simulink model "sampleModel1762_5_sub_sub"  (R2023a)
settings: Solver=VariableStepAuto  StartTime=0.0  StopTime=10.0  RelTol=1e-3
libraries: hdlsllib x1
settings Model: Creator=user1  LastModifiedBy=user1

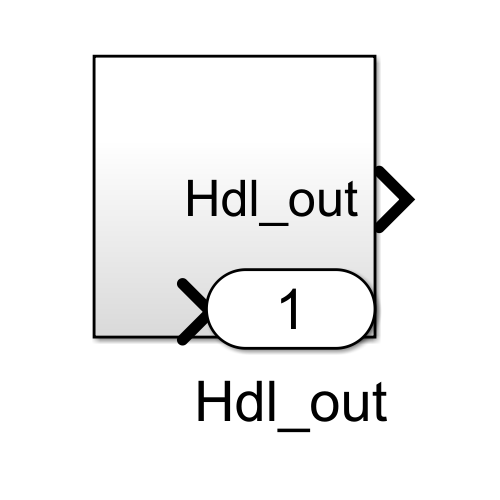
[thumbnail: Simulink's stored preview of the top-level diagram]
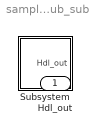
== system sampleModel1762_5_sub_sub ==
  Subsystem : Subsystem
  Hdl_out : Outport  OutDataTypeStr=uint8

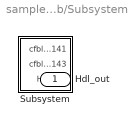
== system sampleModel1762_5_sub_sub/Subsystem ==
  Subsystem : Subsystem
  Hdl_out : Outport  OutDataTypeStr=uint8

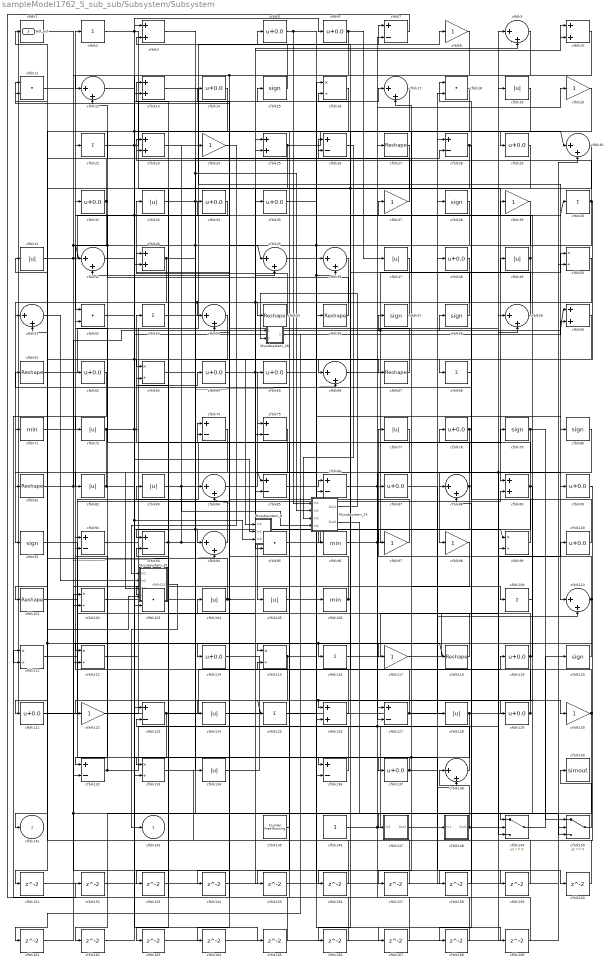
== system sampleModel1762_5_sub_sub/Subsystem/Subsystem ==
  Mysubsystem_23 : Subsystem  TreatAsAtomicUnit=on  RTWFcnName=Mysubsystem_23
      settings: RTWFcnNameOpts=User specified  RTWFileNameOpts=Use function name
  Mysubsystem_28 : Subsystem  TreatAsAtomicUnit=on  RTWFcnName=Mysubsystem_28
      settings: RTWFcnNameOpts=User specified  RTWFileNameOpts=Use function name
  Mysubsystem_35 : Subsystem  TreatAsAtomicUnit=on  RTWFcnName=Mysubsystem_35
      settings: RTWFcnNameOpts=User specified  RTWFileNameOpts=Use function name
  Mysubsystem_8 : Subsystem  TreatAsAtomicUnit=on  RTWFcnName=Mysubsystem_8
      settings: RTWFcnNameOpts=User specified  RTWFileNameOpts=Use function name
  cfblk{1,71,96,106} (4 alike) : MinMax  OutDataTypeStr=uint8
  cfblk{3,10,13,23,25,43,60,89,126} (9 alike) : Sum  OutDataTypeStr=uint8
  cfblk{5..6,14,29,32,34..35,48,62,64..65,78,87,90,100,114,119,121,129,137} (20 alike) : Bias  Bias=0.0  SaturateOnIntegerOverflow=off
  cfblk{27,55..56,61,67,81,101,118} (8 alike) : Reshape
  cfblk{16,50,63,99,102,111..112,115,133} (9 alike) : Product  Inputs=*/  OutDataTypeStr=uint8  RndMeth=Zero  SaturateOnIntegerOverflow=on
  cfblk{11,18,52,95,103} (5 alike) : DotProduct  OutDataTypeStr=uint8
  cfblk{19,33,41,47,49,72,77,82..83,104..105,124,128,134} (14 alike) : Abs  OutDataTypeStr=uint8  SaturateOnIntegerOverflow=off
  cfblk{2,22,40,53,68,109,116,125} (8 alike) : Sum  Inputs=+  OutDataTypeStr=uint8
  cfblk{9,12,17,30,42,45..46,51,54,59,66,84,88,94,110,138} (16 alike) : Sum  Inputs=|++  OutDataTypeStr=uint8
  cfblk{8,20,24,37,39,97..98,117,122,130} (10 alike) : Gain  OutDataTypeStr=uint8
  cfblk{15,38,57..58,79..80,91,120} (8 alike) : Signum
  cfblk{7,26,28,74..75,85..86,92..93,123,127,132,136} (13 alike) : Sum  Inputs=+-  OutDataTypeStr=uint8
  cfblk140 : ToWorkspace  VariableName=simout  SaveFormat=Timeseries  SampleTime=-1
  cfblk145 : hdlsllib/Sources/Counter Free-Running  NumBits=16  tsamp=-1
  cfblk146 : Constant  OutDataTypeStr=uint8  SampleTime=-1
  cfblk147 : Subsystem
      settings: LibrarySourceBlock=|
      | hdlsllib/Ports &
      | Subsystems/Subsystem
  cfblk148 : Subsystem
      settings: LibrarySourceBlock=|
      | hdlsllib/Ports &
      | Subsystems/Subsystem
  cfblk149 : Switch  OutDataTypeStr=uint8  SaturateOnIntegerOverflow=off  InputSameDT=off
  cfblk150 : Switch  OutDataTypeStr=uint8  SaturateOnIntegerOverflow=off  InputSameDT=off
  cfblk{151..169} (19 alike) : Delay  SampleTime=1
  cfblk141 : Outport  OutDataTypeStr=uint8  VectorParamsAs1DForOutWhenUnconnected=off
  cfblk143 : Outport  Port=2  OutDataTypeStr=uint8  VectorParamsAs1DForOutWhenUnconnected=off
  Hdl_out : Outport  Port=3  OutDataTypeStr=uint8
  wires:
  Mysubsystem_35/1(cfblk143) -> cfblk143/1
  cfblk77/1 -> Mysubsystem_35/3(In3)
  cfblk51/1 -> Mysubsystem_35/2(In2)
  cfblk24/1 -> Mysubsystem_35/1(In1)
  Mysubsystem_28/1(Out1) -> cfblk161/1
  Mysubsystem_23/1(Out1) -> Mysubsystem_28/2(In2)
  Mysubsystem_23/2(Out2) -> cfblk162/1
  cfblk26/1 -> Mysubsystem_23/3(In3)
  cfblk52/1 -> Mysubsystem_8/2(In2)
  cfblk169/1 -> cfblk111/1
  cfblk65/1 -> cfblk169/1
  cfblk168/1 -> cfblk127/1
  cfblk39/1 -> cfblk168/1
  cfblk167/1 -> cfblk93/2
  cfblk125/1 -> cfblk167/1
  cfblk166/1 -> cfblk115/2
  cfblk165/1 -> cfblk54/2
  cfblk164/1 -> cfblk30/2
  cfblk163/1 -> cfblk99/2
  cfblk162/1 -> cfblk123/1
  cfblk161/1 -> cfblk102/1
  cfblk160/1 -> cfblk28/1
  cfblk159/1 -> cfblk3/1
  cfblk158/1 -> cfblk88/2
  cfblk157/1 -> cfblk1/1
  cfblk156/1 -> cfblk25/1
  cfblk155/1 -> cfblk138/2
  cfblk38/1 -> cfblk155/1
  cfblk154/1 -> cfblk46/1
  cfblk153/1 -> cfblk50/2
  cfblk29/1 -> cfblk153/1
  cfblk152/1 -> cfblk85/2
  cfblk7/1 -> cfblk152/1
  cfblk151/1 -> cfblk18/2
  cfblk5/1 -> Mysubsystem_23/1(In1), cfblk130/1
  cfblk15/1 -> cfblk5/1
  cfblk14/1 -> cfblk51/2
  cfblk124/1 -> cfblk106/1
  cfblk37/1 -> cfblk12/2
  cfblk12/1 -> cfblk95/1, Mysubsystem_8/3(In3), cfblk30/1
  cfblk98/1 -> cfblk117/1
  cfblk58/1 -> cfblk17/2
  cfblk8/1 -> cfblk43/2
  cfblk119/1 -> cfblk125/1, cfblk126/1, cfblk23/1, cfblk39/1
  cfblk60/1 -> cfblk112/1
  cfblk129/1 -> cfblk14/1, Hdl_out/1
  cfblk56/1 -> cfblk32/1
  cfblk74/1 -> cfblk141/1
  cfblk6/1 -> cfblk12/1, cfblk47/1
  cfblk49/1 -> cfblk54/1, cfblk103/1, cfblk26/2
  cfblk103/1 -> cfblk58/1
  cfblk45/1 -> cfblk80/1
  cfblk63/1 -> cfblk99/1, cfblk149/2
  cfblk78/1 -> cfblk18/1, cfblk127/2
  cfblk133/1 -> cfblk57/1
  cfblk93/1 -> cfblk84/1, cfblk26/1, cfblk63/2
  cfblk111/1 -> cfblk35/1
  cfblk28/1 -> cfblk68/1, cfblk95/2
  cfblk67/1 -> cfblk11/1
  cfblk101/1 -> cfblk25/2
  cfblk117/1 -> cfblk19/1
  cfblk116/1 -> cfblk59/2
  cfblk130/1 -> cfblk16/2, cfblk163/1
  cfblk71/1 -> cfblk62/1
  cfblk64/1 -> cfblk86/2, cfblk10/1
  cfblk50/1 -> cfblk55/1
  cfblk30/1 -> cfblk124/1
  cfblk81/1 -> Mysubsystem_28/1(In1), cfblk109/1
  cfblk68/1 -> cfblk88/1
  cfblk115/1 -> cfblk28/2, cfblk122/1
  cfblk118/1 -> cfblk83/1
  cfblk82/1 -> cfblk81/1, cfblk94/1
  cfblk46/1 -> cfblk93/1, cfblk75/2
  cfblk145/1 -> cfblk75/1
  cfblk47/1 -> cfblk121/1
  cfblk62/1 -> cfblk111/2
  cfblk43/1 -> cfblk132/2, cfblk137/1
  cfblk112/1 -> cfblk74/2
  cfblk80/1 -> cfblk85/1, cfblk149/3
  cfblk85/1 -> cfblk86/1
  cfblk84/1 -> cfblk65/1
  cfblk128/1 -> cfblk156/1, cfblk157/1, cfblk158/1
  cfblk121/1 -> cfblk89/2
  cfblk10/1 -> cfblk13/2
  cfblk42/1 -> cfblk15/1, cfblk40/1
  cfblk19/1 -> cfblk147/1(In1)
  cfblk22/1 -> cfblk8/1, cfblk165/1
  cfblk147/1(Out1) -> cfblk110/2
  cfblk94/1 -> cfblk13/1
  cfblk90/1 -> cfblk134/1
  cfblk127/1 -> cfblk50/1, cfblk92/1
  cfblk105/1 -> cfblk16/1
  cfblk91/1 -> cfblk148/1(In1)
  cfblk16/1 -> cfblk132/1
  cfblk3/1 -> cfblk45/1, cfblk67/1
  cfblk40/1 -> Mysubsystem_8/1(In1), cfblk126/2, cfblk164/1, cfblk23/2
  cfblk27/1 -> cfblk63/1, cfblk136/1
  cfblk53/1 -> cfblk7/2
  cfblk123/1 -> cfblk48/1, cfblk133/2
  cfblk132/1 -> cfblk38/1, cfblk87/1, cfblk92/2
  cfblk109/1 -> cfblk149/1
  cfblk99/1 -> cfblk61/1
  cfblk86/1 -> cfblk78/1, cfblk90/1
  cfblk92/1 -> cfblk56/1
  cfblk136/1 -> cfblk123/2
  cfblk79/1 -> cfblk98/1, cfblk150/1
  cfblk95/1 -> cfblk97/1
  cfblk106/1 -> cfblk42/2, cfblk166/1
  cfblk1/1 -> cfblk116/1, cfblk118/1, cfblk45/2
  cfblk104/1 -> cfblk9/2, cfblk84/2, cfblk41/1
  cfblk66/1 -> cfblk60/1, cfblk10/2
  cfblk146/1 -> cfblk59/1, cfblk20/1
  cfblk61/1 -> cfblk9/1
  cfblk150/1 -> cfblk140/1
  cfblk20/1 -> cfblk42/1, cfblk72/1
  cfblk23/1 -> Mysubsystem_23/2(In2), cfblk66/2
  cfblk54/1 -> cfblk101/1, cfblk103/2
  cfblk138/1 -> cfblk104/1
  cfblk35/1 -> cfblk46/2, cfblk150/2
  cfblk120/1 -> cfblk114/1
  cfblk148/1(Out1) -> cfblk138/1, cfblk100/1
  cfblk75/1 -> cfblk82/1
  cfblk41/1 -> cfblk34/1, cfblk94/2
  cfblk72/1 -> cfblk64/1, cfblk60/2, cfblk112/2
  cfblk97/1 -> cfblk43/1
  cfblk18/1 -> cfblk66/1
  cfblk87/1 -> cfblk128/1
  cfblk83/1 -> Mysubsystem_23/4(In4), cfblk24/1
  cfblk57/1 -> cfblk51/1
  cfblk55/1 -> cfblk33/1
  cfblk134/1 -> cfblk27/1
  cfblk110/1 -> Mysubsystem_35/4(In4), cfblk151/1, cfblk77/1
  cfblk100/1 -> cfblk74/1
  cfblk102/1 -> cfblk17/1
  cfblk59/1 -> cfblk3/2
  cfblk89/1 -> cfblk53/1, cfblk96/1, cfblk129/1
  cfblk32/1 -> cfblk52/1, cfblk11/2
  cfblk126/1 -> cfblk22/1
  cfblk11/1 -> cfblk150/3, cfblk159/1
  cfblk137/1 -> cfblk133/1, cfblk160/1
  cfblk34/1 -> cfblk2/1
  cfblk33/1 -> cfblk7/1, cfblk136/2
  cfblk96/1 -> cfblk49/1, cfblk79/1
  cfblk149/1 -> cfblk120/1
  cfblk25/1 -> cfblk29/1, cfblk71/1
  cfblk114/1 -> cfblk119/1
  cfblk9/1 -> cfblk102/2, cfblk154/1
  cfblk17/1 -> cfblk115/1
  cfblk13/1 -> cfblk110/1
  cfblk2/1 -> cfblk89/1, cfblk6/1
  cfblk122/1 -> cfblk37/1
  cfblk48/1 -> cfblk91/1
  cfblk88/1 -> cfblk105/1, cfblk52/2

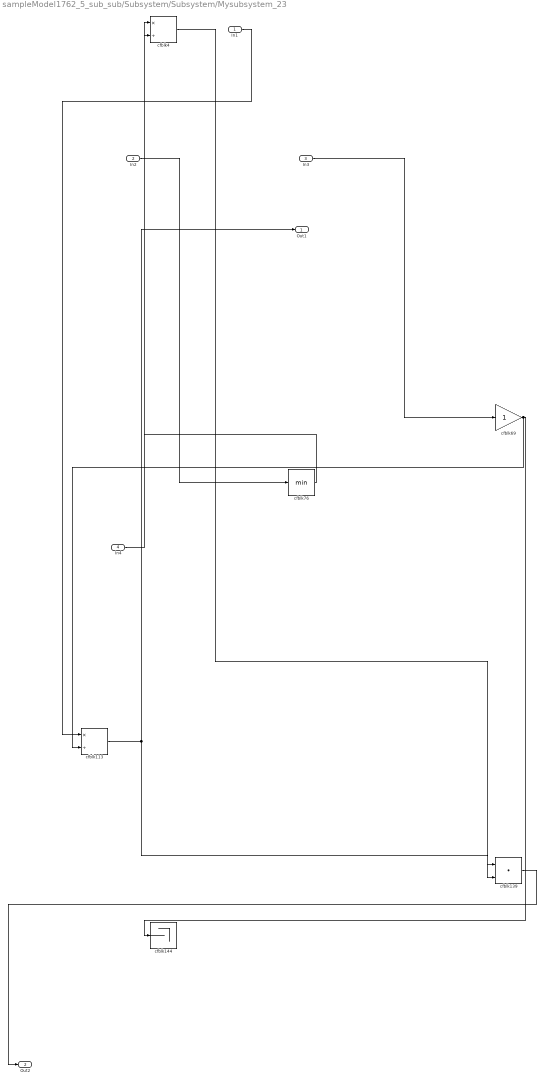
== system sampleModel1762_5_sub_sub/Subsystem/Subsystem/Mysubsystem_23 ==
  In1 : Inport
  In2 : Inport  Port=2
  In3 : Inport  Port=3
  In4 : Inport  Port=4
  cfblk113 : Product  Inputs=*/  RndMeth=Zero  SaturateOnIntegerOverflow=on
  cfblk139 : DotProduct  OutDataTypeStr=Inherit: Inherit via internal rule
  cfblk144 : Terminator
  cfblk4 : Product  Inputs=*/  RndMeth=Zero  SaturateOnIntegerOverflow=on
  cfblk69 : Gain
  cfblk76 : MinMax
  Out1 : Outport
  Out2 : Outport  Port=2
  wires:
  cfblk113/1 -> Out1/1, cfblk139/2
  In2/1 -> cfblk76/1
  cfblk69/1 -> cfblk144/1, cfblk113/2
  In3/1 -> cfblk69/1
  In1/1 -> cfblk113/1
  cfblk4/1 -> cfblk139/1
  cfblk76/1 -> cfblk4/1
  cfblk139/1 -> Out2/1
  In4/1 -> cfblk4/2

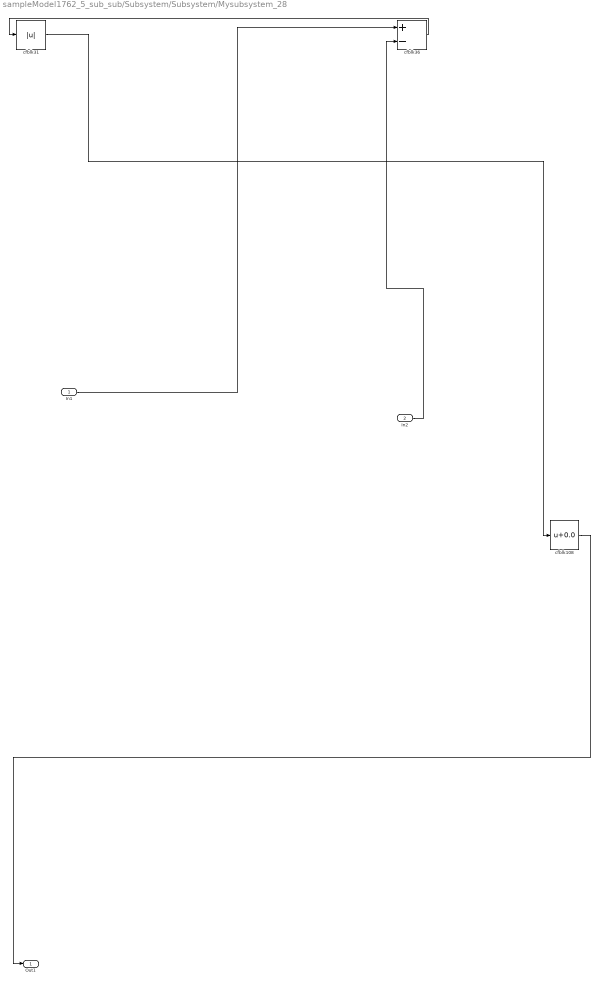
== system sampleModel1762_5_sub_sub/Subsystem/Subsystem/Mysubsystem_28 ==
  In1 : Inport
  In2 : Inport  Port=2
  cfblk108 : Bias  Bias=0.0  SaturateOnIntegerOverflow=off
  cfblk31 : Abs  SaturateOnIntegerOverflow=off
  cfblk36 : Sum  Inputs=+-
  Out1 : Outport
  wires:
  cfblk36/1 -> cfblk31/1
  cfblk31/1 -> cfblk108/1
  In1/1 -> cfblk36/1
  In2/1 -> cfblk36/2
  cfblk108/1 -> Out1/1

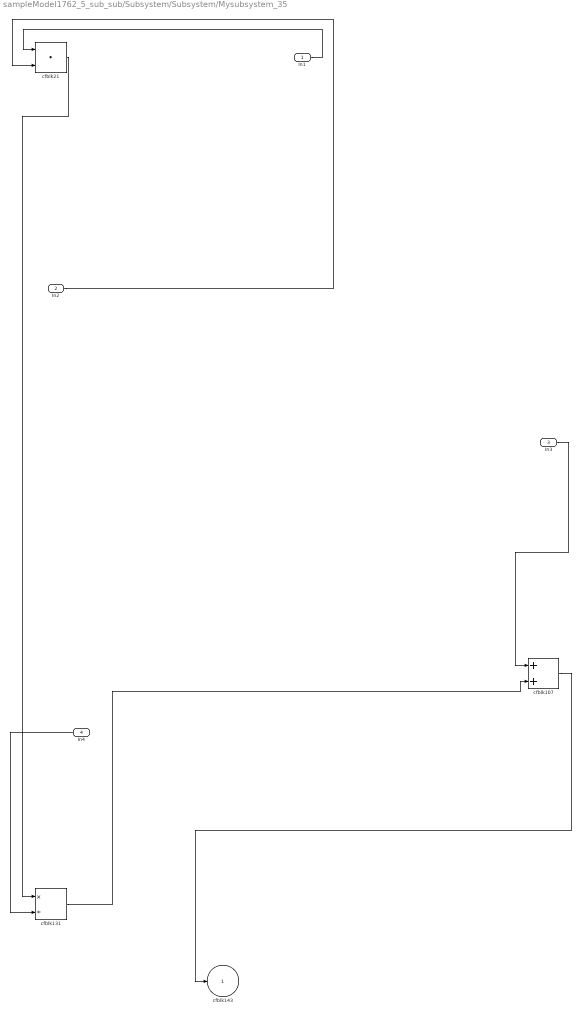
== system sampleModel1762_5_sub_sub/Subsystem/Subsystem/Mysubsystem_35 ==
  In1 : Inport
  In2 : Inport  Port=2
  In3 : Inport  Port=3
  In4 : Inport  Port=4
  cfblk107 : Sum
  cfblk131 : Product  Inputs=*/  RndMeth=Zero  SaturateOnIntegerOverflow=on
  cfblk21 : DotProduct  OutDataTypeStr=Inherit: Inherit via internal rule
  cfblk143 : Outport  VectorParamsAs1DForOutWhenUnconnected=off
  wires:
  In4/1 -> cfblk131/2
  cfblk131/1 -> cfblk107/2
  In2/1 -> cfblk21/2
  In3/1 -> cfblk107/1
  cfblk21/1 -> cfblk131/1
  In1/1 -> cfblk21/1
  cfblk107/1 -> cfblk143/1

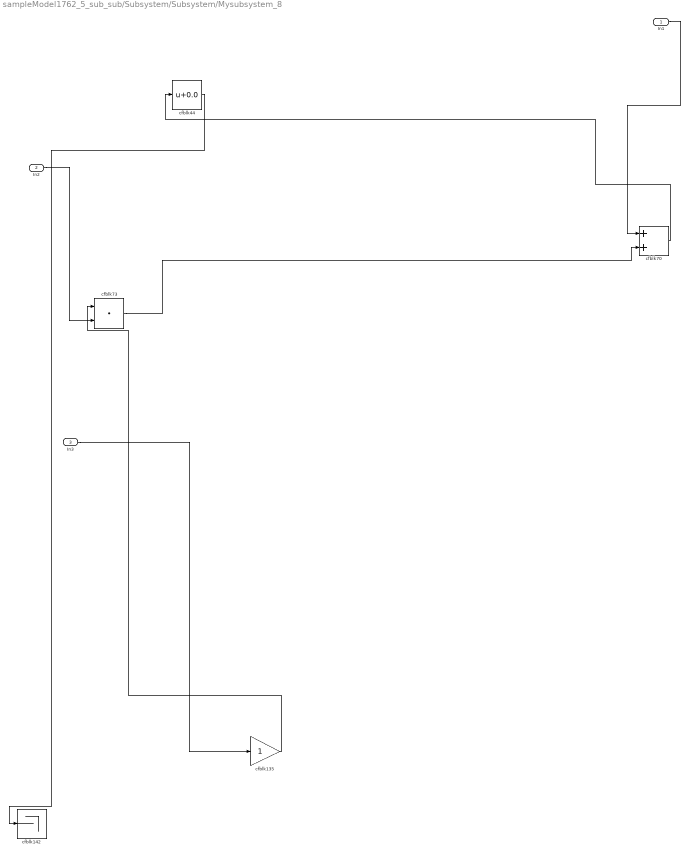
== system sampleModel1762_5_sub_sub/Subsystem/Subsystem/Mysubsystem_8 ==
  In1 : Inport
  In2 : Inport  Port=2
  In3 : Inport  Port=3
  cfblk135 : Gain
  cfblk142 : Terminator
  cfblk44 : Bias  Bias=0.0  SaturateOnIntegerOverflow=off
  cfblk70 : Sum
  cfblk73 : DotProduct  OutDataTypeStr=Inherit: Inherit via internal rule
  wires:
  In2/1 -> cfblk73/2
  cfblk70/1 -> cfblk44/1
  cfblk135/1 -> cfblk73/1
  cfblk73/1 -> cfblk70/2
  In3/1 -> cfblk135/1
  In1/1 -> cfblk70/1
  cfblk44/1 -> cfblk142/1

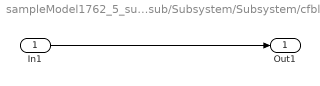
== system sampleModel1762_5_sub_sub/Subsystem/Subsystem/cfblk147 ==
  In1 : Inport
  Out1 : Outport
  wires:
  In1/1 -> Out1/1

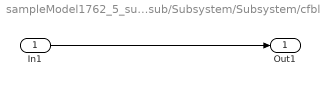
== system sampleModel1762_5_sub_sub/Subsystem/Subsystem/cfblk148 ==
  In1 : Inport
  Out1 : Outport
  wires:
  In1/1 -> Out1/1
